simulink model "nonLinearLoad"  (R2021a)
settings: Solver=VariableStepAuto  StartTime=0.0  StopTime=.04  MaxStep=.0001  RelTol=1e-3
libraries: spsFourierLib x4, spsGroundLib x3, spsRMSLib x2, spsThyristorLib x2, spsACVoltageSourceLib x1, spsCurrentMeasurementLib x1, spsMeanLib x1, spsSeriesRLCBranchLib x1, spsVoltageMeasurementLib x1, spspowerguiLib x1
settings Model: Creator=User  LastModifiedBy=User

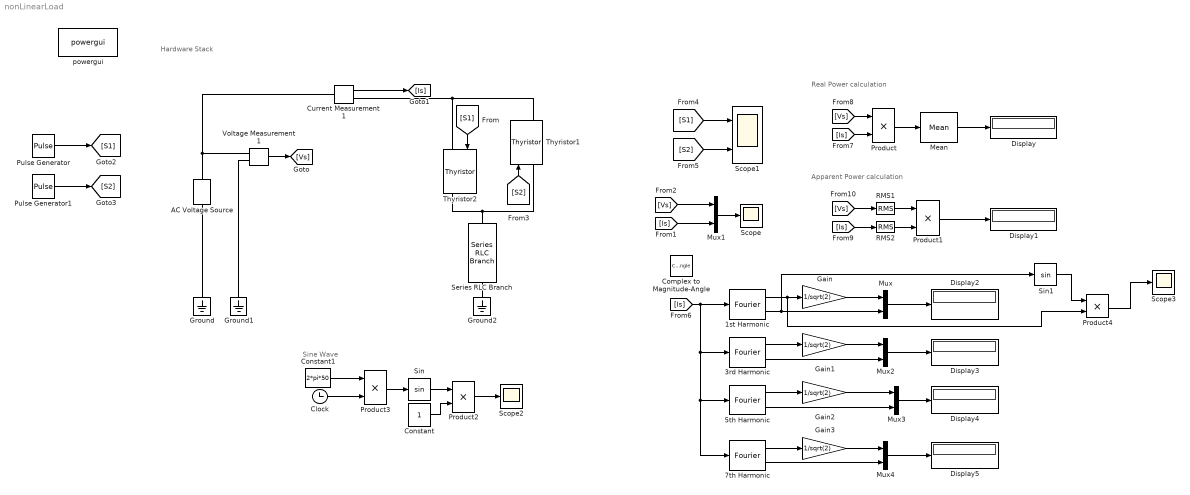
== system nonLinearLoad ==
  note: Sine Wave
  note: Real Power calculation
  note: Hardware Stack
  note: Apparent Power calculation
  1st Harmonic : spsFourierLib/Fourier  Freq=50  n=1  InInit=[0, 0]  Ts=0
      settings: SourceProductBaseCode=PS
  3rd Harmonic : spsFourierLib/Fourier  Freq=50  n=3  InInit=[0, 0]  Ts=0
      settings: SourceProductBaseCode=PS
  5th Harmonic : spsFourierLib/Fourier  Freq=50  n=5  InInit=[0, 0]  Ts=0
      settings: SourceProductBaseCode=PS
  7th Harmonic : spsFourierLib/Fourier  Freq=50  n=7  InInit=[0, 0]  Ts=0
      settings: SourceProductBaseCode=PS
  AC Voltage Source : spsACVoltageSourceLib/AC Voltage Source  Amplitude=310  Phase=0  Frequency=50  SampleTime=0  Measurements=None  BusType=swing  Pref=10e3  Qref=0  Qmin=-inf  Qmax=+inf
  Clock : Clock
  Complex to Magnitude-Angle : ComplexToMagnitudeAngle
  Constant : Constant
  Constant1 : Constant  Value=2*pi*50
  Current Measurement1 : spsCurrentMeasurementLib/Current Measurement  PhasorSimulation=off  OutputType=Complex  PSBequivalent=0
  Display{,1..5} (6 alike) : Display
      Display2 settings: Decimation=2
      Display3 settings: Decimation=2
      Display4 settings: Decimation=2
      Display5 settings: Decimation=2
  Gain{,1..3} (4 alike) : Gain  Gain=1/sqrt(2)
  Ground : spsGroundLib/Ground  LConnTagsString=a
  Ground1 : spsGroundLib/Ground  LConnTagsString=a
  Ground2 : spsGroundLib/Ground  LConnTagsString=a
  Mean : spsMeanLib/Mean  Freq=50  Vinit=0  Ts=0
  Mux{,1..4} (5 alike) : Mux  Inputs=2
  Product{,1..4} (5 alike) : Product
  Pulse Generator : DiscretePulseGenerator  PulseType=Time based  Period=.02  PulseWidth=5  PhaseDelay=90/(2*180*50)
  Pulse Generator1 : DiscretePulseGenerator  PulseType=Time based  Period=1/50  PulseWidth=5  PhaseDelay=90/(2*180*50) +.01
  RMS1 : spsRMSLib/RMS  TrueRMS=on  Freq=50  RMSInit=0  Ts=0
  RMS2 : spsRMSLib/RMS  TrueRMS=on  Freq=50  RMSInit=0  Ts=0
  Scope : Scope
  Scope1 : Scope  NumInputPorts=2
  Scope2 : Scope
  Scope3 : Scope
  Series RLC Branch : spsSeriesRLCBranchLib/Series RLC Branch  LConnTagsString=__new0  RConnTagsString=__new0  BranchType=R  Resistance=10  Inductance=1e-3  SetiL0=off  InitialCurrent=0  Capacitance=1e-6  Setx0=off  InitialVoltage=0  Measurements=None
  Sin : Trigonometry
  Sin1 : Trigonometry
  Thyristor1 : spsThyristorLib/Thyristor  Ron=0.001  Lon=0  Vf=0.8  IC=0  Rs=500  Cs=250e-9  Measurements=on
  Thyristor2 : spsThyristorLib/Thyristor  Ron=0.001  Lon=0  Vf=0.8  IC=0  Rs=500  Cs=250e-9  Measurements=on
  Voltage Measurement1 : spsVoltageMeasurementLib/Voltage Measurement  PhasorSimulation=off  OutputType=Complex  PSBequivalent=0
  powergui : spspowerguiLib/powergui  Priority=1  SimulationMode=Continuous  SampleTime=50e-6  frequency=60  Iterations=50  frequencyindice=50  Pbase=100e6  ErrMax=1e-4  UnitsV=kV  UnitsW=MW  buscounter=0  FunctionMessages=off  echomessages=off  EnableUseOfTLC=off  CurrentSourceSwitches=off  DisableSnubberDevices=on  DisableRonSwitches=on  DisableVfSwitches=on  DisplayEquations=off  AutomaticDiscreteSolvers=off  SolverType=Tustin/Backward Euler (TBE)  Interpol=off  ExternalGateDelay=off  methode=off  Ts=100  x0status=blocks  SPID=on  SwTol=0  HookPort=off  NonlinearTolerance=1e-4  nMaxIteration=100  ContinueOnMaxIteration=off  RestoreLinks=warning  ResistiveCurrentMeasurement=off  Frange=[0:2:500]  Ylog=off  Xlog=on  ShowGrid=off  save=off  variable=ZData  structure=0  ZoomFFT=off  StartTime=0.0  cycles=1  DisplayStyle=1  fundamental=60  FreqAxis=off  MaxFrequency=1000  frequencyindicesteady=1  RmsSteady=1  display=off
  wires:
  Voltage Measurement1/1 -> [Vs]
  Current Measurement1/1 -> [Is]
  Mux1/1 -> Scope/1
  [Vs] -> Mux1/1
  [Is] -> Mux1/2
  Pulse Generator/1 -> [S1]
  Pulse Generator1/1 -> [S2]
  [S1] -> Thyristor2/1
  [S2] -> Thyristor1/1
  [S1] -> Scope1/1
  [S2] -> Scope1/2
  [Is] -> 3rd Harmonic/1, 7th Harmonic/1, 5th Harmonic/1, 1st Harmonic/1
  [Vs] -> Product/1
  [Is] -> Product/2
  Product/1 -> Mean/1
  Mean/1 -> Display/1
  Product1/1 -> Display1/1
  [Is] -> RMS2/1
  [Vs] -> RMS1/1
  RMS1/1 -> Product1/1
  RMS2/1 -> Product1/2
  1st Harmonic/1 -> Product4/2, Gain/1
  Mux/1 -> Display2/1
  Gain/1 -> Mux/1
  1st Harmonic/2 -> Sin1/1, Mux/2
  3rd Harmonic/2 -> Mux2/2
  Gain1/1 -> Mux2/1
  Mux2/1 -> Display3/1
  3rd Harmonic/1 -> Gain1/1
  5th Harmonic/1 -> Gain2/1
  Mux3/1 -> Display4/1
  Gain2/1 -> Mux3/1
  5th Harmonic/2 -> Mux3/2
  7th Harmonic/2 -> Mux4/2
  Gain3/1 -> Mux4/1
  Mux4/1 -> Display5/1
  7th Harmonic/1 -> Gain3/1
  Sin/1 -> Product2/1
  Constant/1 -> Product2/2
  Constant1/1 -> Product3/1
  Clock/1 -> Product3/2
  Product3/1 -> Sin/1
  Product2/1 -> Scope2/1
  Sin1/1 -> Product4/1
  Product4/1 -> Scope3/1
  connections:
  Ground/LConn1 -- AC Voltage Source/LConn1
  Voltage Measurement1/LConn1 -- AC Voltage Source/RConn1 -- Current Measurement1/LConn1
  Ground1/LConn1 -- Voltage Measurement1/LConn2
  Thyristor2/RConn1 -- Thyristor1/LConn1 -- Series RLC Branch/LConn1
  Ground2/LConn1 -- Series RLC Branch/RConn1
  Current Measurement1/RConn1 -- Thyristor1/RConn1 -- Thyristor2/LConn1
